simulink model "Model_3_1"  (R2021a)
settings: Solver=VariableStepAuto  StartTime=0.0  StopTime=10  RelTol=1e-3
InitFcn:
  | bx=0; %25
  | bl=0; %50
  | bc=0.01;
  | 
  | ml=2; %2
  | 
  | mc=0.5;
  | M2=0.5;
  | 
  | mt=5;
  | g=9.81;
  | l_ref=0.1;
  | l_ini=1;
  | l=l_ini;
  | x_ref=1; %5 3
  | n1=1; %5
  | n2=1;
  | 
  | L_2=0;  %chieu dai day nang ha
  | 
  | theta1_ini=0*pi/180;
  | theta2_ini=0*pi/180;  %2*pi/180
  | 
  | L_tai=0.2;
  | %ADRC' s parameter caculation
  | %b0 = (1)/(mc+mt+ml);
  | b0=(ml+mc)/(mt*mc+2*ml*mc+mt*ml+ml^2+mc^2); %Enhanced-coupling
  | %k_ESO = 100;
  | k_ESO = 100;
  | T_set  = 3; %5; 3
  | 
  | s_cl = -5.85/T_set;
  | Kp   = s_cl^2;
  | Kd   = -2*s_cl;
  | 
  | s_ESO = k_ESO*s_cl;
  | l1        = -3*s_ESO;
  | l2        = 3*( s_ESO)^2;
  | l3        = -(s_ESO)^3;
  | 
  | %b1 = (mt+mc)/(mc*ml +mc*mt+ml*mt);
  | b1=1/(ml+mc);
  | k_ESO1 =100; %100
  | T_set1  = 3;   %3
  | s_cl1 = -5.85/T_set1;
  | Kp1   = s_cl1^2;
  | Kd1   = -2*s_cl1;
  | 
  | s_ESO1 = k_ESO1*s_cl1;
  | l11        = -3*s_ESO1;
  | l21        = 3*( s_ESO1)^2;
  | l31        = -(s_ESO1)^3;
  | 
  | 
  | %L1=l_ini;
  | L11=0.55;
  | L2=0.1;
  | m1=2;
  | %m2=M2;
  | m=5;
  | ... (+39 lines)
libraries: neural x1137, simulink x36, simulink_extras x4
(part 3 of 45)

== system Model_3_1/3_1_theta1 bang 0 n1=1; n2=1 2/LT_2bo_2 ==
  ref_ZV : Inport
  In2 : Inport  Port=2
  Bo1_LT_1 : Subsystem
      mask help: Radial Basis Network
      mask Display: e = 0.06;c1 = [120 150 230]/255;c2 = ([120 150 230]+0)/383;c3 = ([120 150 230]+128)/383;patch([0 1 1 0],[0 0 1 1],c1);patch([0 1 1 1-e 1-e 0+e],[0 0 1 1-e 0+e 0+e],c2);patch([0 0 1 1-e 0+e 0+e],[0 1 1 1-e 1-e 0+e],c3);plot([0 1 1 0 0],[0 0 1 1 0]);fprintf('NNET');port_label('input',1,' Input');port_label('output',1,'Output ');
  Bo2_LT_1 : Subsystem
      mask help: Radial Basis Network
      mask Display: e = 0.06;c1 = [120 150 230]/255;c2 = ([120 150 230]+0)/383;c3 = ([120 150 230]+128)/383;patch([0 1 1 0],[0 0 1 1],c1);patch([0 1 1 1-e 1-e 0+e],[0 0 1 1-e 0+e 0+e],c2);patch([0 0 1 1-e 0+e 0+e],[0 1 1 1-e 1-e 0+e],c3);plot([0 1 1 0 0],[0 0 1 1 0]);fprintf('NNET');port_label('input',1,' Input');port_label('output',1,'Output ');
  Constant3 : Constant  Value=mc
  Demux4 : Demux  Outputs=3
  Demux5 : Demux  Outputs=3
  Display7 : Display
  Display8 : Display
  Mux8 : Mux  Inputs=2
  PSO-ETM5 : Subsystem
  PSO-ETM6 : Subsystem
  ref_ZV1 : Outport
  wires:
  PSO-ETM5/1(Out1) -> PSO-ETM6/1(In1)  "ref_ZV"
  Demux5/1 -> PSO-ETM6/2(Input)
  Demux4/3 -> PSO-ETM5/4(Input2)
  Bo2_LT_1/1(Output) -> Demux5/1, Display8/1
  Mux8/1 -> Bo2_LT_1/1(Input), Bo1_LT_1/1(Input)
  Bo1_LT_1/1(Output) -> Display7/1, Demux4/1
  Demux5/2 -> PSO-ETM6/3(Input1)
  Demux5/3 -> PSO-ETM6/4(Input2)
  Demux4/2 -> PSO-ETM5/3(Input1)
  Demux4/1 -> PSO-ETM5/2(Input)
  Constant3/1 -> Mux8/2
  In2/1 -> Mux8/1
  PSO-ETM6/1(ref) -> ref_ZV1/1  "ref_ZV"
  ref_ZV/1 -> PSO-ETM5/1(In1)

== system Model_3_1/3_1_theta1 bang 0 n1=1; n2=1 2/LT_chi_bo1_1 ==
  ref_ZV : Inport
  In2 : Inport  Port=2
  Bo1_LT_1 : Subsystem
      mask help: Radial Basis Network
      mask Display: e = 0.06;c1 = [120 150 230]/255;c2 = ([120 150 230]+0)/383;c3 = ([120 150 230]+128)/383;patch([0 1 1 0],[0 0 1 1],c1);patch([0 1 1 1-e 1-e 0+e],[0 0 1 1-e 0+e 0+e],c2);patch([0 0 1 1-e 0+e 0+e],[0 1 1 1-e 1-e 0+e],c3);plot([0 1 1 0 0],[0 0 1 1 0]);fprintf('NNET');port_label('input',1,' Input');port_label('output',1,'Output ');
  Constant4 : Constant  Value=mc
  Demux2 : Demux  Outputs=3
  Display1 : Display
  Display2 : Display
  Display3 : Display
  Mux9 : Mux  Inputs=2
  PSO-ETM2 : Subsystem
  ref_ : Outport
  wires:
  Demux2/3 -> Display2/1, PSO-ETM2/4(Input2)
  Constant4/1 -> Mux9/2
  PSO-ETM2/1(ref) -> ref_/1  "ref_"
  Demux2/2 -> Display1/1, PSO-ETM2/3(Input1)
  Bo1_LT_1/1(Output) -> Demux2/1
  Mux9/1 -> Bo1_LT_1/1(Input)
  ref_ZV/1 -> PSO-ETM2/1(In1)
  Demux2/1 -> Display3/1, PSO-ETM2/2(Input)
  In2/1 -> Mux9/1

== system Model_3_1/3_1_theta1 bang 0 n1=1; n2=1 2/LT_chi_bo1_2 ==
  ref_ZV : Inport
  In2 : Inport  Port=2
  Bo1_LT_1 : Subsystem
      mask help: Radial Basis Network
      mask Display: e = 0.06;c1 = [120 150 230]/255;c2 = ([120 150 230]+0)/383;c3 = ([120 150 230]+128)/383;patch([0 1 1 0],[0 0 1 1],c1);patch([0 1 1 1-e 1-e 0+e],[0 0 1 1-e 0+e 0+e],c2);patch([0 0 1 1-e 0+e 0+e],[0 1 1 1-e 1-e 0+e],c3);plot([0 1 1 0 0],[0 0 1 1 0]);fprintf('NNET');port_label('input',1,' Input');port_label('output',1,'Output ');
  Constant4 : Constant  Value=mc
  Demux2 : Demux  Outputs=3
  Display1 : Display
  Display2 : Display
  Display3 : Display
  Mux9 : Mux  Inputs=2
  PSO-ETM2 : Subsystem
  ref_ : Outport
  wires:
  Demux2/3 -> Display2/1, PSO-ETM2/4(Input2)
  Constant4/1 -> Mux9/2
  PSO-ETM2/1(ref) -> ref_/1  "ref_"
  Demux2/2 -> Display1/1, PSO-ETM2/3(Input1)
  Bo1_LT_1/1(Output) -> Demux2/1
  Mux9/1 -> Bo1_LT_1/1(Input)
  ref_ZV/1 -> PSO-ETM2/1(In1)
  Demux2/1 -> Display3/1, PSO-ETM2/2(Input)
  In2/1 -> Mux9/1

== system Model_3_1/3_1_theta1 bang 0 n1=1; n2=1 2/PSO_2bo_fl_1 ==
  ref_ZV : Inport
  In2 : Inport  Port=2
  Bo2_LT_2 : Subsystem
      mask help: Radial Basis Network
      mask Display: e = 0.06;c1 = [120 150 230]/255;c2 = ([120 150 230]+0)/383;c3 = ([120 150 230]+128)/383;patch([0 1 1 0],[0 0 1 1],c1);patch([0 1 1 1-e 1-e 0+e],[0 0 1 1-e 0+e 0+e],c2);patch([0 0 1 1-e 0+e 0+e],[0 1 1 1-e 1-e 0+e],c3);plot([0 1 1 0 0],[0 0 1 1 0]);fprintf('NNET');port_label('input',1,' Input');port_label('output',1,'Output ');
  Co FL : Subsystem
      mask help: Radial Basis Network
      mask Display: e = 0.06;c1 = [120 150 230]/255;c2 = ([120 150 230]+0)/383;c3 = ([120 150 230]+128)/383;patch([0 1 1 0],[0 0 1 1],c1);patch([0 1 1 1-e 1-e 0+e],[0 0 1 1-e 0+e 0+e],c2);patch([0 0 1 1-e 0+e 0+e],[0 1 1 1-e 1-e 0+e],c3);plot([0 1 1 0 0],[0 0 1 1 0]);fprintf('NNET');port_label('input',1,' Input');port_label('output',1,'Output ');
  Constant1 : Constant  Value=mc
  Demux1 : Demux  Outputs=3
  Demux3 : Demux  Outputs=3
  Display11 : Display
  Display13 : Display
  Mux4 : Mux  Inputs=2
  PSO-ETM1 : Subsystem
  PSO-ETM3 : Subsystem
  ref_ZV1 : Outport
  wires:
  Demux1/2 -> PSO-ETM3/3(Input1)
  Demux3/1 -> PSO-ETM1/2(Input)
  Demux1/3 -> PSO-ETM3/4(Input2)
  Demux3/3 -> PSO-ETM1/4(Input2)
  Demux3/2 -> PSO-ETM1/3(Input1)
  Bo2_LT_2/1(Output) -> Display13/1, Demux3/1
  PSO-ETM3/1(ref) -> PSO-ETM1/1(In1)  "ref_"
  Constant1/1 -> Mux4/2
  Mux4/1 -> Bo2_LT_2/1(Input), Co FL/1(Input)
  Co FL/1(Output) -> Display11/1, Demux1/1
  Demux1/1 -> PSO-ETM3/2(Input)
  ref_ZV/1 -> PSO-ETM3/1(In1)
  In2/1 -> Mux4/1
  PSO-ETM1/1(ref) -> ref_ZV1/1  "ref_ZV"

== system Model_3_1/3_1_theta1 bang 0 n1=1; n2=1 2/PSO_2bo_fl_2 ==
  ref_ZV : Inport
  In2 : Inport  Port=2
  Bo2_LT_2 : Subsystem
      mask help: Radial Basis Network
      mask Display: e = 0.06;c1 = [120 150 230]/255;c2 = ([120 150 230]+0)/383;c3 = ([120 150 230]+128)/383;patch([0 1 1 0],[0 0 1 1],c1);patch([0 1 1 1-e 1-e 0+e],[0 0 1 1-e 0+e 0+e],c2);patch([0 0 1 1-e 0+e 0+e],[0 1 1 1-e 1-e 0+e],c3);plot([0 1 1 0 0],[0 0 1 1 0]);fprintf('NNET');port_label('input',1,' Input');port_label('output',1,'Output ');
  Co FL : Subsystem
      mask help: Radial Basis Network
      mask Display: e = 0.06;c1 = [120 150 230]/255;c2 = ([120 150 230]+0)/383;c3 = ([120 150 230]+128)/383;patch([0 1 1 0],[0 0 1 1],c1);patch([0 1 1 1-e 1-e 0+e],[0 0 1 1-e 0+e 0+e],c2);patch([0 0 1 1-e 0+e 0+e],[0 1 1 1-e 1-e 0+e],c3);plot([0 1 1 0 0],[0 0 1 1 0]);fprintf('NNET');port_label('input',1,' Input');port_label('output',1,'Output ');
  Constant1 : Constant  Value=mc
  Demux1 : Demux  Outputs=3
  Demux3 : Demux  Outputs=3
  Display11 : Display
  Display13 : Display
  Mux4 : Mux  Inputs=2
  PSO-ETM1 : Subsystem
  PSO-ETM3 : Subsystem
  ref_ZV1 : Outport
  wires:
  Demux1/2 -> PSO-ETM3/3(Input1)
  Demux3/1 -> PSO-ETM1/2(Input)
  Demux1/3 -> PSO-ETM3/4(Input2)
  Demux3/3 -> PSO-ETM1/4(Input2)
  Demux3/2 -> PSO-ETM1/3(Input1)
  Bo2_LT_2/1(Output) -> Display13/1, Demux3/1
  PSO-ETM3/1(ref) -> PSO-ETM1/1(In1)  "ref_"
  Constant1/1 -> Mux4/2
  Mux4/1 -> Bo2_LT_2/1(Input), Co FL/1(Input)
  Co FL/1(Output) -> Display11/1, Demux1/1
  Demux1/1 -> PSO-ETM3/2(Input)
  ref_ZV/1 -> PSO-ETM3/1(In1)
  In2/1 -> Mux4/1
  PSO-ETM1/1(ref) -> ref_ZV1/1  "ref_ZV"

== system Model_3_1/3_1_theta1 bang 0 n1=1; n2=1 2/PSO_2bo_ko_fl_1 ==
  1 : Inport
  In2 : Inport  Port=2
  Bo2_LT_2 : Subsystem
      mask help: Radial Basis Network
      mask Display: e = 0.06;c1 = [120 150 230]/255;c2 = ([120 150 230]+0)/383;c3 = ([120 150 230]+128)/383;patch([0 1 1 0],[0 0 1 1],c1);patch([0 1 1 1-e 1-e 0+e],[0 0 1 1-e 0+e 0+e],c2);patch([0 0 1 1-e 0+e 0+e],[0 1 1 1-e 1-e 0+e],c3);plot([0 1 1 0 0],[0 0 1 1 0]);fprintf('NNET');port_label('input',1,' Input');port_label('output',1,'Output ');
  Co FL : Subsystem
      mask help: Radial Basis Network
      mask Display: e = 0.06;c1 = [120 150 230]/255;c2 = ([120 150 230]+0)/383;c3 = ([120 150 230]+128)/383;patch([0 1 1 0],[0 0 1 1],c1);patch([0 1 1 1-e 1-e 0+e],[0 0 1 1-e 0+e 0+e],c2);patch([0 0 1 1-e 0+e 0+e],[0 1 1 1-e 1-e 0+e],c3);plot([0 1 1 0 0],[0 0 1 1 0]);fprintf('NNET');port_label('input',1,' Input');port_label('output',1,'Output ');
  Constant7 : Constant  Value=mc
  Demux8 : Demux  Outputs=3
  Demux9 : Demux  Outputs=3
  Display10 : Display
  Display9 : Display
  Mux12 : Mux  Inputs=2
  PSO-ETM7 : Subsystem
  PSO-ETM9 : Subsystem
  ko FL2 : Subsystem
      mask help: Radial Basis Network
      mask Display: e = 0.06;c1 = [120 150 230]/255;c2 = ([120 150 230]+0)/383;c3 = ([120 150 230]+128)/383;patch([0 1 1 0],[0 0 1 1],c1);patch([0 1 1 1-e 1-e 0+e],[0 0 1 1-e 0+e 0+e],c2);patch([0 0 1 1-e 0+e 0+e],[0 1 1 1-e 1-e 0+e],c3);plot([0 1 1 0 0],[0 0 1 1 0]);fprintf('NNET');port_label('input',1,' Input');port_label('output',1,'Output ');
  ko co FL_26.1_1 : Subsystem
      mask help: Radial Basis Network
      mask Display: e = 0.06;c1 = [120 150 230]/255;c2 = ([120 150 230]+0)/383;c3 = ([120 150 230]+128)/383;patch([0 1 1 0],[0 0 1 1],c1);patch([0 1 1 1-e 1-e 0+e],[0 0 1 1-e 0+e 0+e],c2);patch([0 0 1 1-e 0+e 0+e],[0 1 1 1-e 1-e 0+e],c3);plot([0 1 1 0 0],[0 0 1 1 0]);fprintf('NNET');port_label('input',1,' Input');port_label('output',1,'Output ');
  ref_ZV : Outport
  wires:
  Demux9/2 -> PSO-ETM7/3(Input1)
  Constant7/1 -> Mux12/2
  Demux8/3 -> PSO-ETM9/4(Input2)
  Mux12/1 -> ko co FL_26.1_1/1(Input), Bo2_LT_2/1(Input)
  Bo2_LT_2/1(Output) -> Demux9/1, Display10/1
  Demux9/3 -> PSO-ETM7/4(Input2)
  PSO-ETM9/1(ref) -> PSO-ETM7/1(In1)  "ref_"
  Demux8/1 -> PSO-ETM9/2(Input)
  Demux9/1 -> PSO-ETM7/2(Input)
  Demux8/2 -> PSO-ETM9/3(Input1)
  ko co FL_26.1_1/1(Output) -> Display9/1, Demux8/1
  In2/1 -> Mux12/1
  1/1 -> PSO-ETM9/1(In1)
  PSO-ETM7/1(ref) -> ref_ZV/1  "ref_ZV"

== system Model_3_1/3_1_theta1 bang 0 n1=1; n2=1 2/PSO_2bo_ko_fl_2 ==
  1 : Inport
  In2 : Inport  Port=2
  Bo2_LT_2 : Subsystem
      mask help: Radial Basis Network
      mask Display: e = 0.06;c1 = [120 150 230]/255;c2 = ([120 150 230]+0)/383;c3 = ([120 150 230]+128)/383;patch([0 1 1 0],[0 0 1 1],c1);patch([0 1 1 1-e 1-e 0+e],[0 0 1 1-e 0+e 0+e],c2);patch([0 0 1 1-e 0+e 0+e],[0 1 1 1-e 1-e 0+e],c3);plot([0 1 1 0 0],[0 0 1 1 0]);fprintf('NNET');port_label('input',1,' Input');port_label('output',1,'Output ');
  Co FL : Subsystem
      mask help: Radial Basis Network
      mask Display: e = 0.06;c1 = [120 150 230]/255;c2 = ([120 150 230]+0)/383;c3 = ([120 150 230]+128)/383;patch([0 1 1 0],[0 0 1 1],c1);patch([0 1 1 1-e 1-e 0+e],[0 0 1 1-e 0+e 0+e],c2);patch([0 0 1 1-e 0+e 0+e],[0 1 1 1-e 1-e 0+e],c3);plot([0 1 1 0 0],[0 0 1 1 0]);fprintf('NNET');port_label('input',1,' Input');port_label('output',1,'Output ');
  Constant7 : Constant  Value=mc
  Demux8 : Demux  Outputs=3
  Demux9 : Demux  Outputs=3
  Display10 : Display
  Display9 : Display
  Mux12 : Mux  Inputs=2
  PSO-ETM7 : Subsystem
  PSO-ETM9 : Subsystem
  ko FL2 : Subsystem
      mask help: Radial Basis Network
      mask Display: e = 0.06;c1 = [120 150 230]/255;c2 = ([120 150 230]+0)/383;c3 = ([120 150 230]+128)/383;patch([0 1 1 0],[0 0 1 1],c1);patch([0 1 1 1-e 1-e 0+e],[0 0 1 1-e 0+e 0+e],c2);patch([0 0 1 1-e 0+e 0+e],[0 1 1 1-e 1-e 0+e],c3);plot([0 1 1 0 0],[0 0 1 1 0]);fprintf('NNET');port_label('input',1,' Input');port_label('output',1,'Output ');
  ko co FL_26.1_1 : Subsystem
      mask help: Radial Basis Network
      mask Display: e = 0.06;c1 = [120 150 230]/255;c2 = ([120 150 230]+0)/383;c3 = ([120 150 230]+128)/383;patch([0 1 1 0],[0 0 1 1],c1);patch([0 1 1 1-e 1-e 0+e],[0 0 1 1-e 0+e 0+e],c2);patch([0 0 1 1-e 0+e 0+e],[0 1 1 1-e 1-e 0+e],c3);plot([0 1 1 0 0],[0 0 1 1 0]);fprintf('NNET');port_label('input',1,' Input');port_label('output',1,'Output ');
  ref_ZV : Outport
  wires:
  Demux9/2 -> PSO-ETM7/3(Input1)
  Constant7/1 -> Mux12/2
  Demux8/3 -> PSO-ETM9/4(Input2)
  Mux12/1 -> ko co FL_26.1_1/1(Input), Bo2_LT_2/1(Input)
  Bo2_LT_2/1(Output) -> Demux9/1, Display10/1
  Demux9/3 -> PSO-ETM7/4(Input2)
  PSO-ETM9/1(ref) -> PSO-ETM7/1(In1)  "ref_"
  Demux8/1 -> PSO-ETM9/2(Input)
  Demux9/1 -> PSO-ETM7/2(Input)
  Demux8/2 -> PSO-ETM9/3(Input1)
  ko co FL_26.1_1/1(Output) -> Display9/1, Demux8/1
  In2/1 -> Mux12/1
  1/1 -> PSO-ETM9/1(In1)
  PSO-ETM7/1(ref) -> ref_ZV/1  "ref_ZV"

== system Model_3_1/3_1_theta1 bang 0 n1=1; n2=1 2/PSO_chi_bo1_1 ==
  1 : Inport
  In2 : Inport  Port=2
  Constant6 : Constant  Value=mc
  Demux7 : Demux  Outputs=3
  Display6 : Display
  Mux11 : Mux  Inputs=2
  PSO-ETM8 : Subsystem
  ko FL2 : Subsystem
      mask help: Radial Basis Network
      mask Display: e = 0.06;c1 = [120 150 230]/255;c2 = ([120 150 230]+0)/383;c3 = ([120 150 230]+128)/383;patch([0 1 1 0],[0 0 1 1],c1);patch([0 1 1 1-e 1-e 0+e],[0 0 1 1-e 0+e 0+e],c2);patch([0 0 1 1-e 0+e 0+e],[0 1 1 1-e 1-e 0+e],c3);plot([0 1 1 0 0],[0 0 1 1 0]);fprintf('NNET');port_label('input',1,' Input');port_label('output',1,'Output ');
  ko co FL_26.1_1 : Subsystem
      mask help: Radial Basis Network
      mask Display: e = 0.06;c1 = [120 150 230]/255;c2 = ([120 150 230]+0)/383;c3 = ([120 150 230]+128)/383;patch([0 1 1 0],[0 0 1 1],c1);patch([0 1 1 1-e 1-e 0+e],[0 0 1 1-e 0+e 0+e],c2);patch([0 0 1 1-e 0+e 0+e],[0 1 1 1-e 1-e 0+e],c3);plot([0 1 1 0 0],[0 0 1 1 0]);fprintf('NNET');port_label('input',1,' Input');port_label('output',1,'Output ');
  ref_ZV : Outport
  wires:
  Demux7/2 -> PSO-ETM8/3(Input1)
  In2/1 -> Mux11/1
  Demux7/3 -> PSO-ETM8/4(Input2)
  Constant6/1 -> Mux11/2
  PSO-ETM8/1(ref) -> ref_ZV/1  "ref_ZV"
  Demux7/1 -> PSO-ETM8/2(Input)
  Mux11/1 -> ko co FL_26.1_1/1(Input)
  ko co FL_26.1_1/1(Output) -> Display6/1, Demux7/1
  1/1 -> PSO-ETM8/1(In1)

== system Model_3_1/3_1_theta1 bang 0 n1=1; n2=1 2/PSO_chi_bo1_2 ==
  1 : Inport
  In2 : Inport  Port=2
  Constant6 : Constant  Value=mc
  Demux7 : Demux  Outputs=3
  Display6 : Display
  Mux11 : Mux  Inputs=2
  PSO-ETM8 : Subsystem
  ko FL2 : Subsystem
      mask help: Radial Basis Network
      mask Display: e = 0.06;c1 = [120 150 230]/255;c2 = ([120 150 230]+0)/383;c3 = ([120 150 230]+128)/383;patch([0 1 1 0],[0 0 1 1],c1);patch([0 1 1 1-e 1-e 0+e],[0 0 1 1-e 0+e 0+e],c2);patch([0 0 1 1-e 0+e 0+e],[0 1 1 1-e 1-e 0+e],c3);plot([0 1 1 0 0],[0 0 1 1 0]);fprintf('NNET');port_label('input',1,' Input');port_label('output',1,'Output ');
  ko co FL_26.1_1 : Subsystem
      mask help: Radial Basis Network
      mask Display: e = 0.06;c1 = [120 150 230]/255;c2 = ([120 150 230]+0)/383;c3 = ([120 150 230]+128)/383;patch([0 1 1 0],[0 0 1 1],c1);patch([0 1 1 1-e 1-e 0+e],[0 0 1 1-e 0+e 0+e],c2);patch([0 0 1 1-e 0+e 0+e],[0 1 1 1-e 1-e 0+e],c3);plot([0 1 1 0 0],[0 0 1 1 0]);fprintf('NNET');port_label('input',1,' Input');port_label('output',1,'Output ');
  ref_ZV : Outport
  wires:
  Demux7/2 -> PSO-ETM8/3(Input1)
  In2/1 -> Mux11/1
  Demux7/3 -> PSO-ETM8/4(Input2)
  Constant6/1 -> Mux11/2
  PSO-ETM8/1(ref) -> ref_ZV/1  "ref_ZV"
  Demux7/1 -> PSO-ETM8/2(Input)
  Mux11/1 -> ko co FL_26.1_1/1(Input)
  ko co FL_26.1_1/1(Output) -> Display6/1, Demux7/1
  1/1 -> PSO-ETM8/1(In1)

== system Model_3_1/3_1_theta1 bang 0 n1=1; n2=1 2/Subsystem1 ==
  e : Inport
  e1 : Inport  Port=2
  Display : Display
  Display12 : Display
  Display16 : Display
  Fitness APS 1 : Subsystem
  Fitness APS 2 : Subsystem
  Gain : Gain  Gain=n1
  Gain19 : Gain  Gain=n2
  Gain20 : Gain  Gain=n2
  Scope : Scope
  Scope71 : Scope
  Scope72 : Scope
  Subtract : Sum
  Subtract1 : Sum  Inputs=+++
  Out1 : Outport
  wires:
  Fitness APS 2/2(MAx) -> Gain20/1, Display16/1, Scope71/1
  Fitness APS 1/2(MAx) -> Display12/1, Gain19/1, Scope72/1
  Subtract/1 -> Gain/1, Display/1, Scope/1
  Gain20/1 -> Subtract1/3
  e/1 -> Fitness APS 1/1(e)
  Gain/1 -> Subtract1/1
  Fitness APS 1/1(IAE) -> Subtract/1
  Gain19/1 -> Subtract1/2
  Fitness APS 2/1(IAE) -> Subtract/2
  e1/1 -> Fitness APS 2/1(e)
  Subtract1/1 -> Out1/1

== system Model_3_1/3_1_theta1 bang 0 n1=1; n2=1 2/Subsystem2 ==
  e : Inport
  e1 : Inport  Port=2
  Display : Display
  Display12 : Display
  Display16 : Display
  Fitness APS 1 : Subsystem
  Fitness APS 2 : Subsystem
  Gain : Gain  Gain=n1
  Gain19 : Gain  Gain=n2
  Gain20 : Gain  Gain=n2
  Scope : Scope
  Scope71 : Scope
  Scope72 : Scope
  Subtract : Sum
  Subtract1 : Sum  Inputs=+++
  Out1 : Outport
  wires:
  Fitness APS 2/2(MAx) -> Gain20/1, Display16/1, Scope71/1
  Fitness APS 1/2(MAx) -> Display12/1, Gain19/1, Scope72/1
  Subtract/1 -> Gain/1, Display/1, Scope/1
  Gain20/1 -> Subtract1/3
  e/1 -> Fitness APS 1/1(e)
  Gain/1 -> Subtract1/1
  Fitness APS 1/1(IAE) -> Subtract/1
  Gain19/1 -> Subtract1/2
  Fitness APS 2/1(IAE) -> Subtract/2
  e1/1 -> Fitness APS 2/1(e)
  Subtract1/1 -> Out1/1

== system Model_3_1/3_1_theta1 bang 0 n1=1; n2=1 2/Subsystem3 ==
  e : Inport
  e1 : Inport  Port=2
  Display : Display
  Display12 : Display
  Display16 : Display
  Fitness APS 1 : Subsystem
  Fitness APS 2 : Subsystem
  Gain : Gain  Gain=n1
  Gain19 : Gain  Gain=n2
  Gain20 : Gain  Gain=n2
  Scope : Scope
  Scope71 : Scope
  Scope72 : Scope
  Subtract : Sum
  Subtract1 : Sum  Inputs=+++
  Out1 : Outport
  wires:
  Fitness APS 2/2(MAx) -> Gain20/1, Display16/1, Scope71/1
  Fitness APS 1/2(MAx) -> Display12/1, Gain19/1, Scope72/1
  Subtract/1 -> Gain/1, Display/1, Scope/1
  Gain20/1 -> Subtract1/3
  e/1 -> Fitness APS 1/1(e)
  Gain/1 -> Subtract1/1
  Fitness APS 1/1(IAE) -> Subtract/1
  Gain19/1 -> Subtract1/2
  Fitness APS 2/1(IAE) -> Subtract/2
  e1/1 -> Fitness APS 2/1(e)
  Subtract1/1 -> Out1/1

== system Model_3_1/3_1_theta1 bang 0 n1=1; n2=1 2/Subsystem4 ==
  e : Inport
  e1 : Inport  Port=2
  Display : Display
  Display12 : Display
  Display16 : Display
  Fitness APS 1 : Subsystem
  Fitness APS 2 : Subsystem
  Gain : Gain  Gain=n1
  Gain19 : Gain  Gain=n2
  Gain20 : Gain  Gain=n2
  Scope : Scope
  Scope71 : Scope
  Scope72 : Scope
  Subtract : Sum
  Subtract1 : Sum  Inputs=+++
  Out1 : Outport
  wires:
  Fitness APS 2/2(MAx) -> Gain20/1, Display16/1, Scope71/1
  Fitness APS 1/2(MAx) -> Display12/1, Gain19/1, Scope72/1
  Subtract/1 -> Gain/1, Display/1, Scope/1
  Gain20/1 -> Subtract1/3
  e/1 -> Fitness APS 1/1(e)
  Gain/1 -> Subtract1/1
  Fitness APS 1/1(IAE) -> Subtract/1
  Gain19/1 -> Subtract1/2
  Fitness APS 2/1(IAE) -> Subtract/2
  e1/1 -> Fitness APS 2/1(e)
  Subtract1/1 -> Out1/1

== system Model_3_1/3_1_theta1 bang 0 n1=1; n2=1 2/Subsystem5 ==
  e : Inport
  e1 : Inport  Port=2
  Display : Display
  Display12 : Display
  Display16 : Display
  Fitness APS 1 : Subsystem
  Fitness APS 2 : Subsystem
  Gain : Gain  Gain=n1
  Gain19 : Gain  Gain=n2
  Gain20 : Gain  Gain=n2
  Scope : Scope
  Scope71 : Scope
  Scope72 : Scope
  Subtract : Sum
  Subtract1 : Sum  Inputs=+++
  Out1 : Outport
  wires:
  Fitness APS 2/2(MAx) -> Gain20/1, Display16/1, Scope71/1
  Fitness APS 1/2(MAx) -> Display12/1, Gain19/1, Scope72/1
  Subtract/1 -> Gain/1, Display/1, Scope/1
  Gain20/1 -> Subtract1/3
  e/1 -> Fitness APS 1/1(e)
  Gain/1 -> Subtract1/1
  Fitness APS 1/1(IAE) -> Subtract/1
  Gain19/1 -> Subtract1/2
  Fitness APS 2/1(IAE) -> Subtract/2
  e1/1 -> Fitness APS 2/1(e)
  Subtract1/1 -> Out1/1

== system Model_3_1/3_1_theta1 bang 0 n1=1; n2=1 2/Subsystem6 ==
  e : Inport
  e1 : Inport  Port=2
  Display : Display
  Display12 : Display
  Display16 : Display
  Fitness APS 1 : Subsystem
  Fitness APS 2 : Subsystem
  Gain : Gain  Gain=n1
  Gain19 : Gain  Gain=n2
  Gain20 : Gain  Gain=n2
  Scope : Scope
  Scope71 : Scope
  Scope72 : Scope
  Subtract : Sum
  Subtract1 : Sum  Inputs=+++
  Out1 : Outport
  wires:
  Fitness APS 2/2(MAx) -> Gain20/1, Display16/1, Scope71/1
  Fitness APS 1/2(MAx) -> Display12/1, Gain19/1, Scope72/1
  Subtract/1 -> Gain/1, Display/1, Scope/1
  Gain20/1 -> Subtract1/3
  e/1 -> Fitness APS 1/1(e)
  Gain/1 -> Subtract1/1
  Fitness APS 1/1(IAE) -> Subtract/1
  Gain19/1 -> Subtract1/2
  Fitness APS 2/1(IAE) -> Subtract/2
  e1/1 -> Fitness APS 2/1(e)
  Subtract1/1 -> Out1/1

== system Model_3_1/3_1_theta1 bang 0 n1=1; n2=1 2/Theta ==
  From Workspace1 : FromWorkspace  VariableName=the2  SampleTime=5e-3
  From Workspace3 : FromWorkspace  VariableName=the1  SampleTime=5e-3
  Out1 : Outport
  Out2 : Outport  Port=2
  wires:
  From Workspace3/1 -> Out1/1
  From Workspace1/1 -> Out2/1

== system Model_3_1/3_1_theta1 bang 0 n1=1; n2=1 2/Theta1 ==
  From Workspace1 : FromWorkspace  VariableName=the2  SampleTime=5e-3
  From Workspace3 : FromWorkspace  VariableName=the1  SampleTime=5e-3
  1 : Outport
  Out2 : Outport  Port=2
  wires:
  From Workspace3/1 -> 1/1
  From Workspace1/1 -> Out2/1

== system Model_3_1/3_1_theta1 bang 0 n1=1; n2=1 2/Theta2 ==
  From Workspace1 : FromWorkspace  VariableName=the2  SampleTime=5e-3
  From Workspace3 : FromWorkspace  VariableName=the1  SampleTime=5e-3
  1 : Outport
  2 : Outport  Port=2
  wires:
  From Workspace3/1 -> 1/1
  From Workspace1/1 -> 2/1

== system Model_3_1/3_1_theta1 bang 0 n1=1; n2=1 2/Theta3 ==
  From Workspace1 : FromWorkspace  VariableName=the2  SampleTime=5e-3
  From Workspace3 : FromWorkspace  VariableName=the1  SampleTime=5e-3
  1 : Outport
  2 : Outport  Port=2
  wires:
  From Workspace3/1 -> 1/1
  From Workspace1/1 -> 2/1

== system Model_3_1/3_1_theta1 bang 0 n1=1; n2=1 2/Theta4 ==
  From Workspace1 : FromWorkspace  VariableName=the2  SampleTime=5e-3
  From Workspace3 : FromWorkspace  VariableName=the1  SampleTime=5e-3
  1 : Outport
  2 : Outport  Port=2
  wires:
  From Workspace3/1 -> 1/1
  From Workspace1/1 -> 2/1

== system Model_3_1/3_1_theta1 bang 0 n1=1; n2=1 2/Theta5 ==
  From Workspace1 : FromWorkspace  VariableName=the2  SampleTime=5e-3
  From Workspace3 : FromWorkspace  VariableName=the1  SampleTime=5e-3
  1 : Outport
  2 : Outport  Port=2
  wires:
  From Workspace3/1 -> 1/1
  From Workspace1/1 -> 2/1

== system Model_3_1/3_1_theta1 bang 0 n1=1; n2=1 2/Theta6 ==
  From Workspace1 : FromWorkspace  VariableName=the2  SampleTime=5e-3
  From Workspace3 : FromWorkspace  VariableName=the1  SampleTime=5e-3
  1 : Outport
  2 : Outport  Port=2
  wires:
  From Workspace3/1 -> 1/1
  From Workspace1/1 -> 2/1

== system Model_3_1/3_1_theta1 bang 0 n1=n2= 1/ADRC 1 ==
  ref : Inport
  x : Inport  Port=2
  Gain : Gain  Gain=Kp
  Gain1 : Gain  Gain=Kd
  Gain2 : Gain  Gain=1/b0
  Observer : Subsystem
  Sum : Sum  Inputs=|+-
  Sum3 : Sum  Inputs=|+-
  Sum4 : Sum  Inputs=|+-
  u : Outport
  wires:
  Sum4/1 -> Gain2/1
  Sum/1 -> Gain/1
  Gain2/1 -> u/1, Observer/1(u)
  x/1 -> Observer/2(x)
  Sum3/1 -> Sum4/1
  Observer/2(x2) -> Gain1/1
  Gain1/1 -> Sum3/2
  Gain/1 -> Sum3/1
  ref/1 -> Sum/1
  Observer/1(x3) -> Sum4/2
  Observer/3(x1) -> Sum/2

== system Model_3_1/3_1_theta1 bang 0 n1=n2= 1/ADRC 10 ==
  ref : Inport
  x : Inport  Port=2
  Gain : Gain  Gain=Kp
  Gain1 : Gain  Gain=Kd
  Gain2 : Gain  Gain=1/b0
  Observer : Subsystem
  Sum : Sum  Inputs=|+-
  Sum3 : Sum  Inputs=|+-
  Sum4 : Sum  Inputs=|+-
  u : Outport
  wires:
  Sum4/1 -> Gain2/1
  Sum/1 -> Gain/1
  Gain2/1 -> u/1, Observer/1(u)
  x/1 -> Observer/2(x)
  Sum3/1 -> Sum4/1
  Observer/2(x2) -> Gain1/1
  Gain1/1 -> Sum3/2
  Gain/1 -> Sum3/1
  ref/1 -> Sum/1
  Observer/1(x3) -> Sum4/2
  Observer/3(x1) -> Sum/2

== system Model_3_1/3_1_theta1 bang 0 n1=n2= 1/ADRC 11 ==
  ref : Inport
  x : Inport  Port=2
  Gain : Gain  Gain=Kp1
  Gain1 : Gain  Gain=Kd1
  Gain2 : Gain  Gain=1/b1
  Observer : Subsystem
  Sum : Sum  Inputs=|+-
  Sum3 : Sum  Inputs=|+-
  Sum4 : Sum  Inputs=|+-
  u : Outport
  wires:
  Sum4/1 -> Gain2/1
  Sum/1 -> Gain/1
  Gain2/1 -> u/1, Observer/1(u)
  x/1 -> Observer/2(x)
  Sum3/1 -> Sum4/1
  Observer/2(x2) -> Gain1/1
  Gain1/1 -> Sum3/2
  Gain/1 -> Sum3/1
  ref/1 -> Sum/1
  Observer/1(x3) -> Sum4/2
  Observer/3(x1) -> Sum/2

== system Model_3_1/3_1_theta1 bang 0 n1=n2= 1/ADRC 12 ==
  ref : Inport
  x : Inport  Port=2
  Gain : Gain  Gain=Kp1
  Gain1 : Gain  Gain=Kd1
  Gain2 : Gain  Gain=1/b1
  Observer : Subsystem
  Sum : Sum  Inputs=|+-
  Sum3 : Sum  Inputs=|+-
  Sum4 : Sum  Inputs=|+-
  u : Outport
  wires:
  Sum4/1 -> Gain2/1
  Sum/1 -> Gain/1
  Gain2/1 -> u/1, Observer/1(u)
  x/1 -> Observer/2(x)
  Sum3/1 -> Sum4/1
  Observer/2(x2) -> Gain1/1
  Gain1/1 -> Sum3/2
  Gain/1 -> Sum3/1
  ref/1 -> Sum/1
  Observer/1(x3) -> Sum4/2
  Observer/3(x1) -> Sum/2

== system Model_3_1/3_1_theta1 bang 0 n1=n2= 1/ADRC 13 ==
  ref : Inport
  x : Inport  Port=2
  Gain : Gain  Gain=Kp1
  Gain1 : Gain  Gain=Kd1
  Gain2 : Gain  Gain=1/b1
  Observer : Subsystem
  Sum : Sum  Inputs=|+-
  Sum3 : Sum  Inputs=|+-
  Sum4 : Sum  Inputs=|+-
  u : Outport
  wires:
  Sum4/1 -> Gain2/1
  Sum/1 -> Gain/1
  Gain2/1 -> u/1, Observer/1(u)
  x/1 -> Observer/2(x)
  Sum3/1 -> Sum4/1
  Observer/2(x2) -> Gain1/1
  Gain1/1 -> Sum3/2
  Gain/1 -> Sum3/1
  ref/1 -> Sum/1
  Observer/1(x3) -> Sum4/2
  Observer/3(x1) -> Sum/2

== system Model_3_1/3_1_theta1 bang 0 n1=n2= 1/ADRC 14 ==
  ref : Inport
  x : Inport  Port=2
  Gain : Gain  Gain=Kp
  Gain1 : Gain  Gain=Kd
  Gain2 : Gain  Gain=1/b0
  Observer : Subsystem
  Sum : Sum  Inputs=|+-
  Sum3 : Sum  Inputs=|+-
  Sum4 : Sum  Inputs=|+-
  u : Outport
  wires:
  Sum4/1 -> Gain2/1
  Sum/1 -> Gain/1
  Gain2/1 -> u/1, Observer/1(u)
  x/1 -> Observer/2(x)
  Sum3/1 -> Sum4/1
  Observer/2(x2) -> Gain1/1
  Gain1/1 -> Sum3/2
  Gain/1 -> Sum3/1
  ref/1 -> Sum/1
  Observer/1(x3) -> Sum4/2
  Observer/3(x1) -> Sum/2

== system Model_3_1/3_1_theta1 bang 0 n1=n2= 1/ADRC 17 ==
  ref : Inport
  x : Inport  Port=2
  Gain : Gain  Gain=Kp
  Gain1 : Gain  Gain=Kd
  Gain2 : Gain  Gain=1/b0
  Observer : Subsystem
  Sum : Sum  Inputs=|+-
  Sum3 : Sum  Inputs=|+-
  Sum4 : Sum  Inputs=|+-
  u : Outport
  wires:
  Sum4/1 -> Gain2/1
  Sum/1 -> Gain/1
  Gain2/1 -> u/1, Observer/1(u)
  x/1 -> Observer/2(x)
  Sum3/1 -> Sum4/1
  Observer/2(x2) -> Gain1/1
  Gain1/1 -> Sum3/2
  Gain/1 -> Sum3/1
  ref/1 -> Sum/1
  Observer/1(x3) -> Sum4/2
  Observer/3(x1) -> Sum/2

== system Model_3_1/3_1_theta1 bang 0 n1=n2= 1/ADRC 18 ==
  ref : Inport
  x : Inport  Port=2
  Gain : Gain  Gain=Kp1
  Gain1 : Gain  Gain=Kd1
  Gain2 : Gain  Gain=1/b1
  Observer : Subsystem
  Sum : Sum  Inputs=|+-
  Sum3 : Sum  Inputs=|+-
  Sum4 : Sum  Inputs=|+-
  u : Outport
  wires:
  Sum4/1 -> Gain2/1
  Sum/1 -> Gain/1
  Gain2/1 -> u/1, Observer/1(u)
  x/1 -> Observer/2(x)
  Sum3/1 -> Sum4/1
  Observer/2(x2) -> Gain1/1
  Gain1/1 -> Sum3/2
  Gain/1 -> Sum3/1
  ref/1 -> Sum/1
  Observer/1(x3) -> Sum4/2
  Observer/3(x1) -> Sum/2

== system Model_3_1/3_1_theta1 bang 0 n1=n2= 1/ADRC 19 ==
  ref : Inport
  x : Inport  Port=2
  Gain : Gain  Gain=Kp
  Gain1 : Gain  Gain=Kd
  Gain2 : Gain  Gain=1/b0
  Observer : Subsystem
  Sum : Sum  Inputs=|+-
  Sum3 : Sum  Inputs=|+-
  Sum4 : Sum  Inputs=|+-
  u : Outport
  wires:
  Sum4/1 -> Gain2/1
  Sum/1 -> Gain/1
  Gain2/1 -> u/1, Observer/1(u)
  x/1 -> Observer/2(x)
  Sum3/1 -> Sum4/1
  Observer/2(x2) -> Gain1/1
  Gain1/1 -> Sum3/2
  Gain/1 -> Sum3/1
  ref/1 -> Sum/1
  Observer/1(x3) -> Sum4/2
  Observer/3(x1) -> Sum/2

== system Model_3_1/3_1_theta1 bang 0 n1=n2= 1/ADRC 2 ==
  ref : Inport
  x : Inport  Port=2
  Gain : Gain  Gain=Kp1
  Gain1 : Gain  Gain=Kd1
  Gain2 : Gain  Gain=1/b1
  Observer : Subsystem
  Sum : Sum  Inputs=|+-
  Sum3 : Sum  Inputs=|+-
  Sum4 : Sum  Inputs=|+-
  u : Outport
  wires:
  Sum4/1 -> Gain2/1
  Sum/1 -> Gain/1
  Gain2/1 -> u/1, Observer/1(u)
  x/1 -> Observer/2(x)
  Sum3/1 -> Sum4/1
  Observer/2(x2) -> Gain1/1
  Gain1/1 -> Sum3/2
  Gain/1 -> Sum3/1
  ref/1 -> Sum/1
  Observer/1(x3) -> Sum4/2
  Observer/3(x1) -> Sum/2

== system Model_3_1/3_1_theta1 bang 0 n1=n2= 1/ADRC 20 ==
  ref : Inport
  x : Inport  Port=2
  Gain : Gain  Gain=Kp1
  Gain1 : Gain  Gain=Kd1
  Gain2 : Gain  Gain=1/b1
  Observer : Subsystem
  Sum : Sum  Inputs=|+-
  Sum3 : Sum  Inputs=|+-
  Sum4 : Sum  Inputs=|+-
  u : Outport
  wires:
  Sum4/1 -> Gain2/1
  Sum/1 -> Gain/1
  Gain2/1 -> u/1, Observer/1(u)
  x/1 -> Observer/2(x)
  Sum3/1 -> Sum4/1
  Observer/2(x2) -> Gain1/1
  Gain1/1 -> Sum3/2
  Gain/1 -> Sum3/1
  ref/1 -> Sum/1
  Observer/1(x3) -> Sum4/2
  Observer/3(x1) -> Sum/2

== system Model_3_1/3_1_theta1 bang 0 n1=n2= 1/ADRC 3 ==
  ref : Inport
  x : Inport  Port=2
  Gain : Gain  Gain=Kp
  Gain1 : Gain  Gain=Kd
  Gain2 : Gain  Gain=1/b0
  Observer : Subsystem
  Sum : Sum  Inputs=|+-
  Sum3 : Sum  Inputs=|+-
  Sum4 : Sum  Inputs=|+-
  u : Outport
  wires:
  Sum4/1 -> Gain2/1
  Sum/1 -> Gain/1
  Gain2/1 -> u/1, Observer/1(u)
  x/1 -> Observer/2(x)
  Sum3/1 -> Sum4/1
  Observer/2(x2) -> Gain1/1
  Gain1/1 -> Sum3/2
  Gain/1 -> Sum3/1
  ref/1 -> Sum/1
  Observer/1(x3) -> Sum4/2
  Observer/3(x1) -> Sum/2

== system Model_3_1/3_1_theta1 bang 0 n1=n2= 1/ADRC 4 ==
  ref : Inport
  x : Inport  Port=2
  Gain : Gain  Gain=Kp1
  Gain1 : Gain  Gain=Kd1
  Gain2 : Gain  Gain=1/b1
  Observer : Subsystem
  Sum : Sum  Inputs=|+-
  Sum3 : Sum  Inputs=|+-
  Sum4 : Sum  Inputs=|+-
  u : Outport
  wires:
  Sum4/1 -> Gain2/1
  Sum/1 -> Gain/1
  Gain2/1 -> u/1, Observer/1(u)
  x/1 -> Observer/2(x)
  Sum3/1 -> Sum4/1
  Observer/2(x2) -> Gain1/1
  Gain1/1 -> Sum3/2
  Gain/1 -> Sum3/1
  ref/1 -> Sum/1
  Observer/1(x3) -> Sum4/2
  Observer/3(x1) -> Sum/2

== system Model_3_1/3_1_theta1 bang 0 n1=n2= 1/ADRC 9 ==
  ref : Inport
  x : Inport  Port=2
  Gain : Gain  Gain=Kp
  Gain1 : Gain  Gain=Kd
  Gain2 : Gain  Gain=1/b0
  Observer : Subsystem
  Sum : Sum  Inputs=|+-
  Sum3 : Sum  Inputs=|+-
  Sum4 : Sum  Inputs=|+-
  u : Outport
  wires:
  Sum4/1 -> Gain2/1
  Sum/1 -> Gain/1
  Gain2/1 -> u/1, Observer/1(u)
  x/1 -> Observer/2(x)
  Sum3/1 -> Sum4/1
  Observer/2(x2) -> Gain1/1
  Gain1/1 -> Sum3/2
  Gain/1 -> Sum3/1
  ref/1 -> Sum/1
  Observer/1(x3) -> Sum4/2
  Observer/3(x1) -> Sum/2

== system Model_3_1/3_1_theta1 bang 0 n1=n2= 1/Bo1_LT_1 ==
  Input : Inport  PortDimensions=2
      mask Display: e = 0.06;c1 = [120 230 180]/255;c2 = ([120 230 180]+0)/(256+128);c3 = ([120 230 180]+128)/(256+128);patch([0 1 1 0],[0 0 1 1],c1);patch([0 1 1 1-e 1-e 0+e],[0 0 1 1-e 0+e 0+e],c2);patch([0 0 1 1-e 0+e 0+e],[0 1 1 1-e 1-e 0+e],c3);plot([0 1 1 0 0],[0 0 1 1 0]);
  Layer 1 : Subsystem
      mask Display: e = 0.06;c1 = [120 150 230]/255;c2 = ([120 150 230]+0)/383;c3 = ([120 150 230]+128)/383;patch([0 1 1 0],[0 0 1 1],c1);patch([0 1 1 1-e 1-e 0+e],[0 0 1 1-e 0+e 0+e],c2);patch([0 0 1 1-e 0+e 0+e],[0 1 1 1-e 1-e 0+e],c3);plot([0 1 1 0 0],[0 0 1 1 0]);
  Layer 2 : Subsystem
      mask Display: e = 0.06;c1 = [120 150 230]/255;c2 = ([120 150 230]+0)/383;c3 = ([120 150 230]+128)/383;patch([0 1 1 0],[0 0 1 1],c1);patch([0 1 1 1-e 1-e 0+e],[0 0 1 1-e 0+e 0+e],c2);patch([0 0 1 1-e 0+e 0+e],[0 1 1 1-e 1-e 0+e],c3);plot([0 1 1 0 0],[0 0 1 1 0]);
  Process Input 1 : Subsystem
      mask Display: e = 0.06;c1 = [120 150 230]/255;c2 = ([120 150 230]+0)/383;c3 = ([120 150 230]+128)/383;patch([0 1 1 0],[0 0 1 1],c1);patch([0 1 1 1-e 1-e 0+e],[0 0 1 1-e 0+e 0+e],c2);patch([0 0 1 1-e 0+e 0+e],[0 1 1 1-e 1-e 0+e],c3);plot([0 1 1 0 0],[0 0 1 1 0]);
  Process Output 1 : Subsystem
      mask Display: e = 0.06;c1 = [120 150 230]/255;c2 = ([120 150 230]+0)/383;c3 = ([120 150 230]+128)/383;patch([0 1 1 0],[0 0 1 1],c1);patch([0 1 1 1-e 1-e 0+e],[0 0 1 1-e 0+e 0+e],c2);patch([0 0 1 1-e 0+e 0+e],[0 1 1 1-e 1-e 0+e],c3);plot([0 1 1 0 0],[0 0 1 1 0]);
  Output : Outport  InitialOutput=[0;0;0]
      mask Display: e = 0.06;c1 = [120 230 180]/255;c2 = ([120 230 180]+0)/(256+128);c3 = ([120 230 180]+128)/(256+128);patch([0 1 1 0],[0 0 1 1],c1);patch([0 1 1 1-e 1-e 0+e],[0 0 1 1-e 0+e 0+e],c2);patch([0 0 1 1-e 0+e 0+e],[0 1 1 1-e 1-e 0+e],c3);plot([0 1 1 0 0],[0 0 1 1 0]);
  wires:
  Input/1 -> Process Input 1/1(x)
  Process Output 1/1(y) -> Output/1
  Process Input 1/1(p) -> Layer 1/1("p{1}")
  Layer 1/1("a{1}") -> [feedback1]
  [feedback1] -> Layer 2/1("a{1} ")
  Layer 2/1("a{2}") -> Process Output 1/1(a)

== system Model_3_1/3_1_theta1 bang 0 n1=n2= 1/Bo1_LT_2 ==
  Input : Inport  PortDimensions=2
      mask Display: e = 0.06;c1 = [120 230 180]/255;c2 = ([120 230 180]+0)/(256+128);c3 = ([120 230 180]+128)/(256+128);patch([0 1 1 0],[0 0 1 1],c1);patch([0 1 1 1-e 1-e 0+e],[0 0 1 1-e 0+e 0+e],c2);patch([0 0 1 1-e 0+e 0+e],[0 1 1 1-e 1-e 0+e],c3);plot([0 1 1 0 0],[0 0 1 1 0]);
  Layer 1 : Subsystem
      mask Display: e = 0.06;c1 = [120 150 230]/255;c2 = ([120 150 230]+0)/383;c3 = ([120 150 230]+128)/383;patch([0 1 1 0],[0 0 1 1],c1);patch([0 1 1 1-e 1-e 0+e],[0 0 1 1-e 0+e 0+e],c2);patch([0 0 1 1-e 0+e 0+e],[0 1 1 1-e 1-e 0+e],c3);plot([0 1 1 0 0],[0 0 1 1 0]);
  Layer 2 : Subsystem
      mask Display: e = 0.06;c1 = [120 150 230]/255;c2 = ([120 150 230]+0)/383;c3 = ([120 150 230]+128)/383;patch([0 1 1 0],[0 0 1 1],c1);patch([0 1 1 1-e 1-e 0+e],[0 0 1 1-e 0+e 0+e],c2);patch([0 0 1 1-e 0+e 0+e],[0 1 1 1-e 1-e 0+e],c3);plot([0 1 1 0 0],[0 0 1 1 0]);
  Process Input 1 : Subsystem
      mask Display: e = 0.06;c1 = [120 150 230]/255;c2 = ([120 150 230]+0)/383;c3 = ([120 150 230]+128)/383;patch([0 1 1 0],[0 0 1 1],c1);patch([0 1 1 1-e 1-e 0+e],[0 0 1 1-e 0+e 0+e],c2);patch([0 0 1 1-e 0+e 0+e],[0 1 1 1-e 1-e 0+e],c3);plot([0 1 1 0 0],[0 0 1 1 0]);
  Process Output 1 : Subsystem
      mask Display: e = 0.06;c1 = [120 150 230]/255;c2 = ([120 150 230]+0)/383;c3 = ([120 150 230]+128)/383;patch([0 1 1 0],[0 0 1 1],c1);patch([0 1 1 1-e 1-e 0+e],[0 0 1 1-e 0+e 0+e],c2);patch([0 0 1 1-e 0+e 0+e],[0 1 1 1-e 1-e 0+e],c3);plot([0 1 1 0 0],[0 0 1 1 0]);
  Output : Outport  InitialOutput=[0;0;0]
      mask Display: e = 0.06;c1 = [120 230 180]/255;c2 = ([120 230 180]+0)/(256+128);c3 = ([120 230 180]+128)/(256+128);patch([0 1 1 0],[0 0 1 1],c1);patch([0 1 1 1-e 1-e 0+e],[0 0 1 1-e 0+e 0+e],c2);patch([0 0 1 1-e 0+e 0+e],[0 1 1 1-e 1-e 0+e],c3);plot([0 1 1 0 0],[0 0 1 1 0]);
  wires:
  Input/1 -> Process Input 1/1(x)
  Process Output 1/1(y) -> Output/1
  Process Input 1/1(p) -> Layer 1/1("p{1}")
  Layer 1/1("a{1}") -> [feedback1]
  [feedback1] -> Layer 2/1("a{1} ")
  Layer 2/1("a{2}") -> Process Output 1/1(a)

== system Model_3_1/3_1_theta1 bang 0 n1=n2= 1/Bo2_LT_1 ==
  Input : Inport  PortDimensions=2
      mask Display: e = 0.06;c1 = [120 230 180]/255;c2 = ([120 230 180]+0)/(256+128);c3 = ([120 230 180]+128)/(256+128);patch([0 1 1 0],[0 0 1 1],c1);patch([0 1 1 1-e 1-e 0+e],[0 0 1 1-e 0+e 0+e],c2);patch([0 0 1 1-e 0+e 0+e],[0 1 1 1-e 1-e 0+e],c3);plot([0 1 1 0 0],[0 0 1 1 0]);
  Layer 1 : Subsystem
      mask Display: e = 0.06;c1 = [120 150 230]/255;c2 = ([120 150 230]+0)/383;c3 = ([120 150 230]+128)/383;patch([0 1 1 0],[0 0 1 1],c1);patch([0 1 1 1-e 1-e 0+e],[0 0 1 1-e 0+e 0+e],c2);patch([0 0 1 1-e 0+e 0+e],[0 1 1 1-e 1-e 0+e],c3);plot([0 1 1 0 0],[0 0 1 1 0]);
  Layer 2 : Subsystem
      mask Display: e = 0.06;c1 = [120 150 230]/255;c2 = ([120 150 230]+0)/383;c3 = ([120 150 230]+128)/383;patch([0 1 1 0],[0 0 1 1],c1);patch([0 1 1 1-e 1-e 0+e],[0 0 1 1-e 0+e 0+e],c2);patch([0 0 1 1-e 0+e 0+e],[0 1 1 1-e 1-e 0+e],c3);plot([0 1 1 0 0],[0 0 1 1 0]);
  Process Input 1 : Subsystem
      mask Display: e = 0.06;c1 = [120 150 230]/255;c2 = ([120 150 230]+0)/383;c3 = ([120 150 230]+128)/383;patch([0 1 1 0],[0 0 1 1],c1);patch([0 1 1 1-e 1-e 0+e],[0 0 1 1-e 0+e 0+e],c2);patch([0 0 1 1-e 0+e 0+e],[0 1 1 1-e 1-e 0+e],c3);plot([0 1 1 0 0],[0 0 1 1 0]);
  Process Output 1 : Subsystem
      mask Display: e = 0.06;c1 = [120 150 230]/255;c2 = ([120 150 230]+0)/383;c3 = ([120 150 230]+128)/383;patch([0 1 1 0],[0 0 1 1],c1);patch([0 1 1 1-e 1-e 0+e],[0 0 1 1-e 0+e 0+e],c2);patch([0 0 1 1-e 0+e 0+e],[0 1 1 1-e 1-e 0+e],c3);plot([0 1 1 0 0],[0 0 1 1 0]);
  Output : Outport  InitialOutput=[0;0;0]
      mask Display: e = 0.06;c1 = [120 230 180]/255;c2 = ([120 230 180]+0)/(256+128);c3 = ([120 230 180]+128)/(256+128);patch([0 1 1 0],[0 0 1 1],c1);patch([0 1 1 1-e 1-e 0+e],[0 0 1 1-e 0+e 0+e],c2);patch([0 0 1 1-e 0+e 0+e],[0 1 1 1-e 1-e 0+e],c3);plot([0 1 1 0 0],[0 0 1 1 0]);
  wires:
  Input/1 -> Process Input 1/1(x)
  Process Output 1/1(y) -> Output/1
  Process Input 1/1(p) -> Layer 1/1("p{1}")
  Layer 1/1("a{1}") -> [feedback1]
  [feedback1] -> Layer 2/1("a{1} ")
  Layer 2/1("a{2}") -> Process Output 1/1(a)

== system Model_3_1/3_1_theta1 bang 0 n1=n2= 1/Bo2_LT_2 ==
  Input : Inport  PortDimensions=2
      mask Display: e = 0.06;c1 = [120 230 180]/255;c2 = ([120 230 180]+0)/(256+128);c3 = ([120 230 180]+128)/(256+128);patch([0 1 1 0],[0 0 1 1],c1);patch([0 1 1 1-e 1-e 0+e],[0 0 1 1-e 0+e 0+e],c2);patch([0 0 1 1-e 0+e 0+e],[0 1 1 1-e 1-e 0+e],c3);plot([0 1 1 0 0],[0 0 1 1 0]);
  Layer 1 : Subsystem
      mask Display: e = 0.06;c1 = [120 150 230]/255;c2 = ([120 150 230]+0)/383;c3 = ([120 150 230]+128)/383;patch([0 1 1 0],[0 0 1 1],c1);patch([0 1 1 1-e 1-e 0+e],[0 0 1 1-e 0+e 0+e],c2);patch([0 0 1 1-e 0+e 0+e],[0 1 1 1-e 1-e 0+e],c3);plot([0 1 1 0 0],[0 0 1 1 0]);
  Layer 2 : Subsystem
      mask Display: e = 0.06;c1 = [120 150 230]/255;c2 = ([120 150 230]+0)/383;c3 = ([120 150 230]+128)/383;patch([0 1 1 0],[0 0 1 1],c1);patch([0 1 1 1-e 1-e 0+e],[0 0 1 1-e 0+e 0+e],c2);patch([0 0 1 1-e 0+e 0+e],[0 1 1 1-e 1-e 0+e],c3);plot([0 1 1 0 0],[0 0 1 1 0]);
  Process Input 1 : Subsystem
      mask Display: e = 0.06;c1 = [120 150 230]/255;c2 = ([120 150 230]+0)/383;c3 = ([120 150 230]+128)/383;patch([0 1 1 0],[0 0 1 1],c1);patch([0 1 1 1-e 1-e 0+e],[0 0 1 1-e 0+e 0+e],c2);patch([0 0 1 1-e 0+e 0+e],[0 1 1 1-e 1-e 0+e],c3);plot([0 1 1 0 0],[0 0 1 1 0]);
  Process Output 1 : Subsystem
      mask Display: e = 0.06;c1 = [120 150 230]/255;c2 = ([120 150 230]+0)/383;c3 = ([120 150 230]+128)/383;patch([0 1 1 0],[0 0 1 1],c1);patch([0 1 1 1-e 1-e 0+e],[0 0 1 1-e 0+e 0+e],c2);patch([0 0 1 1-e 0+e 0+e],[0 1 1 1-e 1-e 0+e],c3);plot([0 1 1 0 0],[0 0 1 1 0]);
  Output : Outport  InitialOutput=[0;0;0]
      mask Display: e = 0.06;c1 = [120 230 180]/255;c2 = ([120 230 180]+0)/(256+128);c3 = ([120 230 180]+128)/(256+128);patch([0 1 1 0],[0 0 1 1],c1);patch([0 1 1 1-e 1-e 0+e],[0 0 1 1-e 0+e 0+e],c2);patch([0 0 1 1-e 0+e 0+e],[0 1 1 1-e 1-e 0+e],c3);plot([0 1 1 0 0],[0 0 1 1 0]);
  wires:
  Input/1 -> Process Input 1/1(x)
  Process Output 1/1(y) -> Output/1
  Process Input 1/1(p) -> Layer 1/1("p{1}")
  Layer 1/1("a{1}") -> [feedback1]
  [feedback1] -> Layer 2/1("a{1} ")
  Layer 2/1("a{2}") -> Process Output 1/1(a)

== system Model_3_1/3_1_theta1 bang 0 n1=n2= 1/Bo2_LT_3 ==
  Input : Inport  PortDimensions=2
      mask Display: e = 0.06;c1 = [120 230 180]/255;c2 = ([120 230 180]+0)/(256+128);c3 = ([120 230 180]+128)/(256+128);patch([0 1 1 0],[0 0 1 1],c1);patch([0 1 1 1-e 1-e 0+e],[0 0 1 1-e 0+e 0+e],c2);patch([0 0 1 1-e 0+e 0+e],[0 1 1 1-e 1-e 0+e],c3);plot([0 1 1 0 0],[0 0 1 1 0]);
  Layer 1 : Subsystem
      mask Display: e = 0.06;c1 = [120 150 230]/255;c2 = ([120 150 230]+0)/383;c3 = ([120 150 230]+128)/383;patch([0 1 1 0],[0 0 1 1],c1);patch([0 1 1 1-e 1-e 0+e],[0 0 1 1-e 0+e 0+e],c2);patch([0 0 1 1-e 0+e 0+e],[0 1 1 1-e 1-e 0+e],c3);plot([0 1 1 0 0],[0 0 1 1 0]);
  Layer 2 : Subsystem
      mask Display: e = 0.06;c1 = [120 150 230]/255;c2 = ([120 150 230]+0)/383;c3 = ([120 150 230]+128)/383;patch([0 1 1 0],[0 0 1 1],c1);patch([0 1 1 1-e 1-e 0+e],[0 0 1 1-e 0+e 0+e],c2);patch([0 0 1 1-e 0+e 0+e],[0 1 1 1-e 1-e 0+e],c3);plot([0 1 1 0 0],[0 0 1 1 0]);
  Process Input 1 : Subsystem
      mask Display: e = 0.06;c1 = [120 150 230]/255;c2 = ([120 150 230]+0)/383;c3 = ([120 150 230]+128)/383;patch([0 1 1 0],[0 0 1 1],c1);patch([0 1 1 1-e 1-e 0+e],[0 0 1 1-e 0+e 0+e],c2);patch([0 0 1 1-e 0+e 0+e],[0 1 1 1-e 1-e 0+e],c3);plot([0 1 1 0 0],[0 0 1 1 0]);
  Process Output 1 : Subsystem
      mask Display: e = 0.06;c1 = [120 150 230]/255;c2 = ([120 150 230]+0)/383;c3 = ([120 150 230]+128)/383;patch([0 1 1 0],[0 0 1 1],c1);patch([0 1 1 1-e 1-e 0+e],[0 0 1 1-e 0+e 0+e],c2);patch([0 0 1 1-e 0+e 0+e],[0 1 1 1-e 1-e 0+e],c3);plot([0 1 1 0 0],[0 0 1 1 0]);
  Output : Outport  InitialOutput=[0;0;0]
      mask Display: e = 0.06;c1 = [120 230 180]/255;c2 = ([120 230 180]+0)/(256+128);c3 = ([120 230 180]+128)/(256+128);patch([0 1 1 0],[0 0 1 1],c1);patch([0 1 1 1-e 1-e 0+e],[0 0 1 1-e 0+e 0+e],c2);patch([0 0 1 1-e 0+e 0+e],[0 1 1 1-e 1-e 0+e],c3);plot([0 1 1 0 0],[0 0 1 1 0]);
  wires:
  Input/1 -> Process Input 1/1(x)
  Process Output 1/1(y) -> Output/1
  Process Input 1/1(p) -> Layer 1/1("p{1}")
  Layer 1/1("a{1}") -> [feedback1]
  [feedback1] -> Layer 2/1("a{1} ")
  Layer 2/1("a{2}") -> Process Output 1/1(a)

== system Model_3_1/3_1_theta1 bang 0 n1=n2= 1/Co FL ==
  Input : Inport  PortDimensions=2
      mask Display: e = 0.06;c1 = [120 230 180]/255;c2 = ([120 230 180]+0)/(256+128);c3 = ([120 230 180]+128)/(256+128);patch([0 1 1 0],[0 0 1 1],c1);patch([0 1 1 1-e 1-e 0+e],[0 0 1 1-e 0+e 0+e],c2);patch([0 0 1 1-e 0+e 0+e],[0 1 1 1-e 1-e 0+e],c3);plot([0 1 1 0 0],[0 0 1 1 0]);
  Layer 1 : Subsystem
      mask Display: e = 0.06;c1 = [120 150 230]/255;c2 = ([120 150 230]+0)/383;c3 = ([120 150 230]+128)/383;patch([0 1 1 0],[0 0 1 1],c1);patch([0 1 1 1-e 1-e 0+e],[0 0 1 1-e 0+e 0+e],c2);patch([0 0 1 1-e 0+e 0+e],[0 1 1 1-e 1-e 0+e],c3);plot([0 1 1 0 0],[0 0 1 1 0]);
  Layer 2 : Subsystem
      mask Display: e = 0.06;c1 = [120 150 230]/255;c2 = ([120 150 230]+0)/383;c3 = ([120 150 230]+128)/383;patch([0 1 1 0],[0 0 1 1],c1);patch([0 1 1 1-e 1-e 0+e],[0 0 1 1-e 0+e 0+e],c2);patch([0 0 1 1-e 0+e 0+e],[0 1 1 1-e 1-e 0+e],c3);plot([0 1 1 0 0],[0 0 1 1 0]);
  Process Input 1 : Subsystem
      mask Display: e = 0.06;c1 = [120 150 230]/255;c2 = ([120 150 230]+0)/383;c3 = ([120 150 230]+128)/383;patch([0 1 1 0],[0 0 1 1],c1);patch([0 1 1 1-e 1-e 0+e],[0 0 1 1-e 0+e 0+e],c2);patch([0 0 1 1-e 0+e 0+e],[0 1 1 1-e 1-e 0+e],c3);plot([0 1 1 0 0],[0 0 1 1 0]);
  Process Output 1 : Subsystem
      mask Display: e = 0.06;c1 = [120 150 230]/255;c2 = ([120 150 230]+0)/383;c3 = ([120 150 230]+128)/383;patch([0 1 1 0],[0 0 1 1],c1);patch([0 1 1 1-e 1-e 0+e],[0 0 1 1-e 0+e 0+e],c2);patch([0 0 1 1-e 0+e 0+e],[0 1 1 1-e 1-e 0+e],c3);plot([0 1 1 0 0],[0 0 1 1 0]);
  Output : Outport  InitialOutput=[0;0;0]
      mask Display: e = 0.06;c1 = [120 230 180]/255;c2 = ([120 230 180]+0)/(256+128);c3 = ([120 230 180]+128)/(256+128);patch([0 1 1 0],[0 0 1 1],c1);patch([0 1 1 1-e 1-e 0+e],[0 0 1 1-e 0+e 0+e],c2);patch([0 0 1 1-e 0+e 0+e],[0 1 1 1-e 1-e 0+e],c3);plot([0 1 1 0 0],[0 0 1 1 0]);
  wires:
  Input/1 -> Process Input 1/1(x)
  Process Output 1/1(y) -> Output/1
  Process Input 1/1(p) -> Layer 1/1("p{1}")
  Layer 1/1("a{1}") -> [feedback1]
  [feedback1] -> Layer 2/1("a{1} ")
  Layer 2/1("a{2}") -> Process Output 1/1(a)

== system Model_3_1/3_1_theta1 bang 0 n1=n2= 1/Co bx, bl, bc-1 ==
  Fx : Inport
  Fl : Inport  Port=2
  Add : Sum
  Constant : Constant  Value=-(m1+mc)*g
  Constant1 : Constant  Value=mc
  Constant2 : Constant  Value=L_tai
  Constant3 : Constant  Value=bx
  Constant4 : Constant  Value=bl
  Constant5 : Constant  Value=bc
  Crane : MATLAB Function  TreatAsAtomicUnit=on
  Integrator{,1,3,5,7} (5 alike) : Integrator
  Integrator2 : Integrator  InitialCondition=l
  Integrator4 : Integrator  InitialCondition=theta1_ini
  Integrator6 : Integrator  InitialCondition=theta2_ini
  Scope{1..5} (5 alike) : Scope
  x : Outport
  l : Outport  Port=2
  the1 : Outport  Port=3
  the2 : Outport  Port=4
  wires:
  Integrator5/1 -> [x6]
  Integrator2/1 -> Scope4/1, l/1, [x3]
  Integrator1/1 -> [x2]
  Integrator/1 -> x/1, [x1]
  Integrator3/1 -> [x4]
  Add/1 -> Crane/9(Fl), Scope1/1
  Integrator6/1 -> Scope2/1, the2/1, [x7]
  Integrator7/1 -> [x8]
  Crane/1(dx1) -> Integrator/1
  Crane/2(dx2) -> Integrator1/1
  Crane/3(dx3) -> Integrator2/1
  Crane/4(dx4) -> Integrator3/1
  Crane/5(dx5) -> Integrator4/1
  Crane/6(dx6) -> Integrator5/1
  Crane/7(dx7) -> Integrator6/1
  Crane/8(dx8) -> Integrator7/1
  Fx/1 -> Crane/8(Fx)
  Constant1/1 -> Crane/10(m2)
  [x2] -> Crane/1(d1x)
  [x3] -> Crane/2(l1)
  [x4] -> Crane/3(d1l1)
  [x5] -> Crane/4(the1)
  [x6] -> Crane/5(d1the1)
  [x7] -> Crane/6(the2)
  [x8] -> Crane/7(d1the2)
  Integrator4/1 -> Scope3/1, the1/1, [x5]
  Fl/1 -> Add/2
  [x1] -> Scope5/1
  Constant/1 -> Add/1
  Constant2/1 -> Crane/11(l2)
  Constant3/1 -> Crane/12(bx)
  Constant4/1 -> Crane/13(bl)
  Constant5/1 -> Crane/14(bc)

== system Model_3_1/3_1_theta1 bang 0 n1=n2= 1/ETM2 ==
  ref_ETm4 : Inport
  ETM1 : Subsystem
  ETM4 : Subsystem
  ref1 : Scope
  ref2 : Scope
  ref3 : Scope
  ref_ETM4 : Outport
  wires:
  ETM1/1(Out1) -> ref2/1, ETM4/1(In1)  "ref_ZV"
  ETM4/1(Out1) -> ref3/1, ref_ETM4/1  "ref_ZV"
  ref_ETm4/1 -> ref1/1, ETM1/1(In1)

== system Model_3_1/3_1_theta1 bang 0 n1=n2= 1/Ko co bx, bl, bc-1 ==
  Fx : Inport
  Fl : Inport  Port=2
  Add : Sum
  Constant : Constant  Value=-(m1+mc)*g
  Constant1 : Constant  Value=mc
  Constant2 : Constant  Value=L_tai
  Crane : MATLAB Function  TreatAsAtomicUnit=on
  Integrator{,1,3,5,7} (5 alike) : Integrator
  Integrator2 : Integrator  InitialCondition=l
  Integrator4 : Integrator  InitialCondition=theta1_ini
  Integrator6 : Integrator  InitialCondition=theta2_ini
  Scope{1..5} (5 alike) : Scope
  x : Outport
  l : Outport  Port=2
  the1 : Outport  Port=3
  the2 : Outport  Port=4
  wires:
  Integrator5/1 -> [x6]
  Integrator2/1 -> Scope4/1, l/1, [x3]
  Integrator1/1 -> [x2]
  Integrator/1 -> x/1, [x1]
  Integrator3/1 -> [x4]
  Add/1 -> Scope1/1, Crane/9(Fl)
  Integrator6/1 -> Scope2/1, the2/1, [x7]
  Integrator7/1 -> [x8]
  Crane/1(dx1) -> Integrator/1
  Crane/2(dx2) -> Integrator1/1
  Crane/3(dx3) -> Integrator2/1
  Crane/4(dx4) -> Integrator3/1
  Crane/5(dx5) -> Integrator4/1
  Crane/6(dx6) -> Integrator5/1
  Crane/7(dx7) -> Integrator6/1
  Crane/8(dx8) -> Integrator7/1
  Fx/1 -> Crane/8(Fx)
  Constant1/1 -> Crane/10(m2)
  [x2] -> Crane/1(d1x)
  [x3] -> Crane/2(l1)
  [x4] -> Crane/3(d1l1)
  [x5] -> Crane/4(the1)
  [x6] -> Crane/5(d1the1)
  [x7] -> Crane/6(the2)
  [x8] -> Crane/7(d1the2)
  Integrator4/1 -> Scope3/1, the1/1, [x5]
  Fl/1 -> Add/2
  [x1] -> Scope5/1
  Constant/1 -> Add/1
  Constant2/1 -> Crane/11(l2)

== system Model_3_1/3_1_theta1 bang 0 n1=n2= 1/Ko co bx, bl, bc-2 ==
  Fx : Inport
  Fl : Inport  Port=2
  Add : Sum
  Constant : Constant  Value=-(m1+mc)*g
  Constant1 : Constant  Value=mc
  Constant2 : Constant  Value=L_tai
  Crane : MATLAB Function  TreatAsAtomicUnit=on
  Integrator{,1,3,5,7} (5 alike) : Integrator
  Integrator2 : Integrator  InitialCondition=l
  Integrator4 : Integrator  InitialCondition=theta1_ini
  Integrator6 : Integrator  InitialCondition=theta2_ini
  Scope{1..5} (5 alike) : Scope
  x : Outport
  l : Outport  Port=2
  the1 : Outport  Port=3
  the2 : Outport  Port=4
  wires:
  Integrator5/1 -> [x6]
  Integrator2/1 -> Scope4/1, l/1, [x3]
  Integrator1/1 -> [x2]
  Integrator/1 -> x/1, [x1]
  Integrator3/1 -> [x4]
  Add/1 -> Scope1/1, Crane/9(Fl)
  Integrator6/1 -> Scope2/1, the2/1, [x7]
  Integrator7/1 -> [x8]
  Crane/1(dx1) -> Integrator/1
  Crane/2(dx2) -> Integrator1/1
  Crane/3(dx3) -> Integrator2/1
  Crane/4(dx4) -> Integrator3/1
  Crane/5(dx5) -> Integrator4/1
  Crane/6(dx6) -> Integrator5/1
  Crane/7(dx7) -> Integrator6/1
  Crane/8(dx8) -> Integrator7/1
  Fx/1 -> Crane/8(Fx)
  Constant1/1 -> Crane/10(m2)
  [x2] -> Crane/1(d1x)
  [x3] -> Crane/2(l1)
  [x4] -> Crane/3(d1l1)
  [x5] -> Crane/4(the1)
  [x6] -> Crane/5(d1the1)
  [x7] -> Crane/6(the2)
  [x8] -> Crane/7(d1the2)
  Integrator4/1 -> Scope3/1, the1/1, [x5]
  Fl/1 -> Add/2
  [x1] -> Scope5/1
  Constant/1 -> Add/1
  Constant2/1 -> Crane/11(l2)

== system Model_3_1/3_1_theta1 bang 0 n1=n2= 1/Ko co bx, bl, bc-3 ==
  Fx : Inport
  Fl : Inport  Port=2
  Add : Sum
  Constant : Constant  Value=-(m1+mc)*g
  Constant1 : Constant  Value=mc
  Constant2 : Constant  Value=L_tai
  Crane : MATLAB Function  TreatAsAtomicUnit=on
  Integrator{,1,3,5,7} (5 alike) : Integrator
  Integrator2 : Integrator  InitialCondition=l
  Integrator4 : Integrator  InitialCondition=theta1_ini
  Integrator6 : Integrator  InitialCondition=theta2_ini
  Scope{1..5} (5 alike) : Scope
  x : Outport
  l : Outport  Port=2
  the1 : Outport  Port=3
  the2 : Outport  Port=4
  wires:
  Integrator5/1 -> [x6]
  Integrator2/1 -> Scope4/1, l/1, [x3]
  Integrator1/1 -> [x2]
  Integrator/1 -> x/1, [x1]
  Integrator3/1 -> [x4]
  Add/1 -> Scope1/1, Crane/9(Fl)
  Integrator6/1 -> Scope2/1, the2/1, [x7]
  Integrator7/1 -> [x8]
  Crane/1(dx1) -> Integrator/1
  Crane/2(dx2) -> Integrator1/1
  Crane/3(dx3) -> Integrator2/1
  Crane/4(dx4) -> Integrator3/1
  Crane/5(dx5) -> Integrator4/1
  Crane/6(dx6) -> Integrator5/1
  Crane/7(dx7) -> Integrator6/1
  Crane/8(dx8) -> Integrator7/1
  Fx/1 -> Crane/8(Fx)
  Constant1/1 -> Crane/10(m2)
  [x2] -> Crane/1(d1x)
  [x3] -> Crane/2(l1)
  [x4] -> Crane/3(d1l1)
  [x5] -> Crane/4(the1)
  [x6] -> Crane/5(d1the1)
  [x7] -> Crane/6(the2)
  [x8] -> Crane/7(d1the2)
  Integrator4/1 -> Scope3/1, the1/1, [x5]
  Fl/1 -> Add/2
  [x1] -> Scope5/1
  Constant/1 -> Add/1
  Constant2/1 -> Crane/11(l2)
